simulink model "trapezi_simulink"  (R2022b)
settings: Solver=VariableStepAuto  StartTime=0.0  StopTime=10.0  RelTol=1e-3
libraries: fuzblock x1, simulink_extras x1
settings Model: Creator=Σάββας  LastModifiedBy=Σάββας

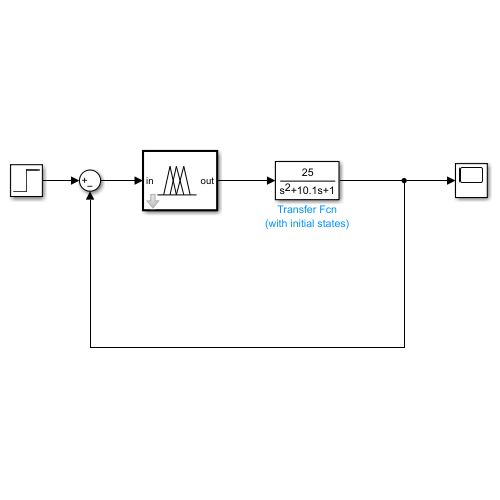
[thumbnail: Simulink's stored preview of the top-level diagram]
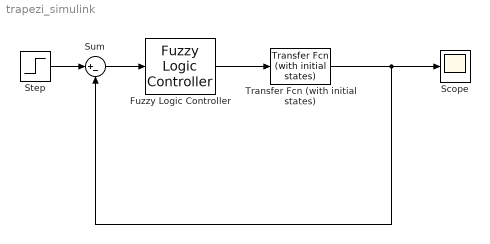
== system trapezi_simulink ==
  Fuzzy Logic Controller : fuzblock/Fuzzy Logic  Controller  FIS='tipper.fis'  OutputSampleNumber=101  DataType=double  FuzzifiedInputs=off  RuleFiringStrengths=off  RuleOutputs=off  AggregatedOutputs=off  SimulateUsing=Interpreted execution  OutOfRangeInputValueMessage=warning  NoRuleFiredMessage=warning  EmptyOutputFuzzySetMessage=warning
  Scope : Scope
  Step : Step  SampleTime=0
  Sum : Sum  Inputs=|+-
  Transfer Fcn (with initial states) : simulink_extras/Additional Linear/Transfer Fcn (with initial states)  N=[25]  D="[1 10.1  1]"  X0=.5
  wires:
  Step/1 -> Sum/1
  Sum/1 -> Fuzzy Logic Controller/1
  Transfer Fcn (with initial states)/1 -> Scope/1, Sum/2
  Fuzzy Logic Controller/1 -> Transfer Fcn (with initial states)/1
